simulink model "TheoryVsDataMdl"  (R2023b)
settings: Solver=VariableStepAuto  StartTime=0.0  StopTime=10.0  RelTol=1e-3
undefined symbols (not defined in the file or in its folder): V_tf_d, V_tf_n
settings Model: Creator=joeashton  LastModifiedBy=joeashton

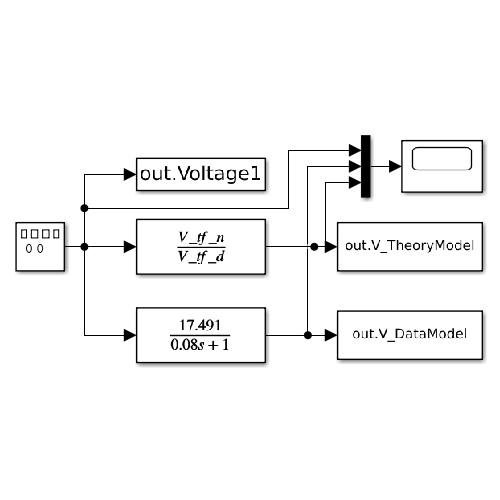
[thumbnail: Simulink's stored preview of the top-level diagram]
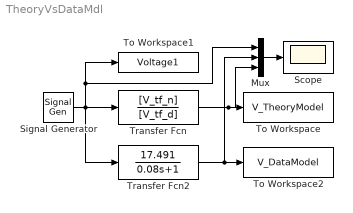
== system TheoryVsDataMdl ==
  Mux : Mux  Inputs=3
  Scope : Scope
  Signal Generator : SignalGenerator  WaveForm=square  Amplitude=2  Frequency=0.4
  To Workspace : ToWorkspace  VariableName=V_TheoryModel  SaveFormat=Timeseries  SampleTime=-1
  To Workspace1 : ToWorkspace  VariableName=Voltage1  SaveFormat=Timeseries  SampleTime=-1
  To Workspace2 : ToWorkspace  VariableName=V_DataModel  SaveFormat=Timeseries  SampleTime=-1
  Transfer Fcn : TransferFcn  Numerator=[V_tf_n]  Denominator=[V_tf_d]
  Transfer Fcn2 : TransferFcn  Numerator=[17.491]  Denominator=[0.08 1]
  wires:
  Transfer Fcn/1 -> Mux/3, To Workspace/1
  Signal Generator/1 -> Transfer Fcn2/1, Transfer Fcn/1, To Workspace1/1, Mux/1
  Mux/1 -> Scope/1
  Transfer Fcn2/1 -> To Workspace2/1, Mux/2
